simulink model "AUV_Model"  (R2023a)
settings: Solver=VariableStepAuto  StartTime=0.0  StopTime=300  FixedStep=0.5  RelTol=1e-3
InitFcn:
  | mdlWks = get_param(gcs,'ModelWorkspace');
  | a = getVariable(mdlWks,'a');
  | b = getVariable(mdlWks,'b');
  | c = getVariable(mdlWks,'c');
StopFcn:
  | figure(2)
  | plot3(Position_Data(1,1),Position_Data(1,2),Position_Data(1,3),'r*')
  | hold on
  | plot3(Position_Data(:,1),Position_Data(:,2),Position_Data(:,3));
  | plot3(Position_Data(end,1),Position_Data(end,2),Position_Data(end,3),'g*');
  | grid on
  | legend('Start Point','Trajectory','End Point')
model workspace (MAT data in the model file):
  a = 0
  b = 1
  c = 1
undefined symbols (not defined in the file or in its folder): sigbuilder_block
libraries: sharedtransform x6, vrlib x6, dspfdesign x6, sim3dlib x3, slpidlib x3, simulink x2, shared6dof x1, aerolibasang x1, aerolibnav x1, sim3dphyssensorlib x1
(part 1 of 2)
settings Model: Creator=yveerall  LastModifiedBy=kellthom
settings SolverCC: AlgebraicLoopSolver=TrustRegion
settings DataIOCC: ReturnWorkspaceOutputs=off
settings DebuggingCC: UnconnectedInputMsg=warning  UnconnectedOutputMsg=warning  UnconnectedLineMsg=warning  ArithmeticOperatorsInVariantConditions=warning
settings ModelReferenceCC: EnableRefExpFcnMdlSchedulingChecks=on
settings SFSimCC: CustomCodeUndefinedFunction=UseInterfaceOnly
settings RTWCC: DLArmComputeVersion=19.05

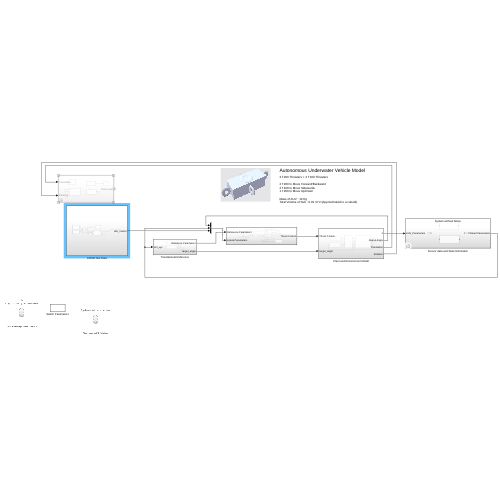
[thumbnail: Simulink's stored preview of the top-level diagram]
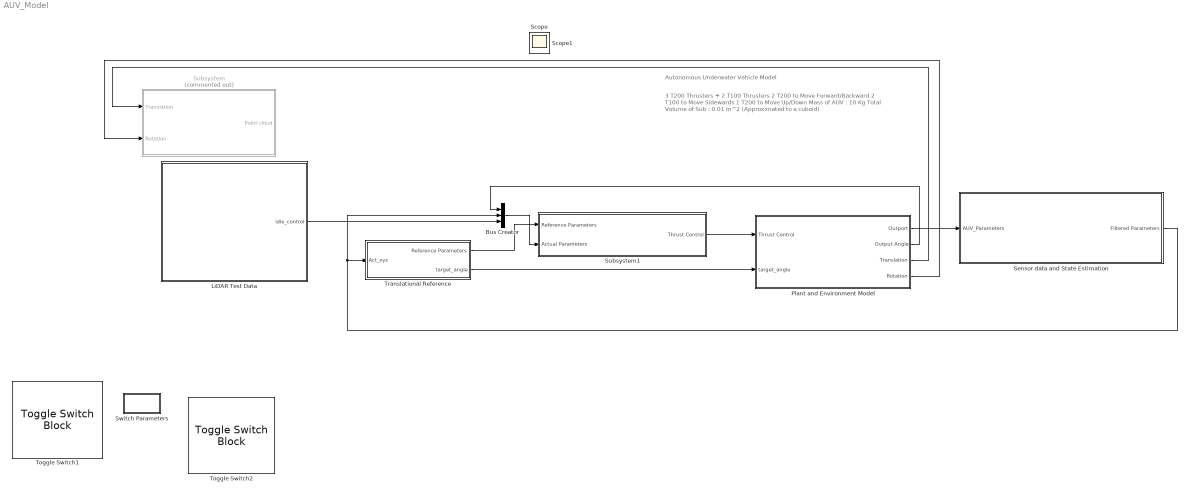
== system AUV_Model ==
  note: Autonomous Underwater Vehicle Model
  note: 3 T200 Thrusters + 2 T100 Thrusters
      |
      | 2 T200 to Move Forward/Backward
      | 2 T100 to Move Sidewards
      | 1 T200 to Move Up/Down
      |
      | Mass of AUV : 10 Kg
      | Total Volume of Sub : 0.01 m^2 (Approximated to a cuboid)
  Bus Creator : BusCreator  Inputs=3
  LiDAR Test Data : Subsystem
  Plant and Environment Model : Subsystem
  Sensor data and State Estimation : Subsystem  Variant=on
  Subsystem : Subsystem  Commented=on
  Subsystem1 : Subsystem
  Switch Parameters : Subsystem
      mask Display: text(0.5, 0.5, 'Switch Parameters', 'horizontalAlignment', 'center')
  Toggle Switch1 : ToggleSwitchBlock
      settings: Values={{'Low Fidelity Simulation', 'High Fidelity Simulation'}, [0 1]}
  Toggle Switch2 : ToggleSwitchBlock
      settings: Values={{'System with Noise', 'System without Noise'}, [0 1]}
  Translational Reference : Subsystem
  Scope : Scope
  Scope1 : Scope
  wires:
  Plant and Environment Model/1(Outport) -> Sensor data and State Estimation/1(AUV_Parameters)
  Sensor data and State Estimation/1(Filtered Parameters) -> Bus Creator/2, Translational Reference/1(Act_xyz)
  Translational Reference/2(target_angle) -> Plant and Environment Model/2(target_angle)
  Plant and Environment Model/4(Rotation) -> Subsystem/2(Rotation)
  Plant and Environment Model/3(Translation) -> Subsystem/1(Translation)
  Plant and Environment Model/2(Output Angle) -> Bus Creator/1
  Subsystem1/1(Thrust Control) -> Plant and Environment Model/1(Thrust Control)
  Translational Reference/1(Reference Parameters) -> Subsystem1/1(Reference Parameters)
  Bus Creator/1 -> Subsystem1/2(Actual Parameters)
  LiDAR Test Data/1(idle_control) -> Bus Creator/3

== system AUV_Model/LiDAR Test Data ==
  Clock : Clock
  Lidar control : MATLAB Function  TreatAsAtomicUnit=on
  MATLAB Function : MATLAB Function  TreatAsAtomicUnit=on
  MATLAB Function1 : MATLAB Function  TreatAsAtomicUnit=on
  Point Cloud Viewer : PointCloudViewer  FigPos=[161 681 522 480]
  Rate Transition : RateTransition  OutPortSampleTime=1
  Scope2 : Scope  NumInputPorts=2
  Switch : Switch  Criteria=u2 > Threshold  Threshold=9  SaturateOnIntegerOverflow=off  InputSameDT=off
  idle_control : Outport
  wires:
  Clock/1 -> Rate Transition/1
  Rate Transition/1 -> Switch/2, Lidar control/2(clock)
  Lidar control/2(state_o) -> Scope2/1
  MATLAB Function1/1(pcloud) -> Switch/3
  Switch/1 -> Point Cloud Viewer/1, Lidar control/1(point_cloud)
  Lidar control/1(idle_control) -> idle_control/1
  MATLAB Function/1(pcloud) -> Switch/1

== system AUV_Model/Plant and Environment Model ==
  Thrust Control : Inport
  target_angle : Inport  Port=2
  Combine Forces and Moments : Subsystem
  Dynamics solver : Subsystem
  Environmental Forces & Moments : Subsystem
  Propulsion Forces & Moments : Subsystem
  Outport : Outport  VectorParamsAs1DForOutWhenUnconnected=off
  Output Angle : Outport  Port=2
  Translation : Outport  Port=3  VectorParamsAs1DForOutWhenUnconnected=off
  Rotation : Outport  Port=4  VectorParamsAs1DForOutWhenUnconnected=off
  wires:
  Thrust Control/1 -> Propulsion Forces & Moments/1(Thrust Control In)
  Propulsion Forces & Moments/1(Propulsion Parameters) -> Combine Forces and Moments/1(Propulsion Parameters)
  Environmental Forces & Moments/1(Environment Parameters) -> Combine Forces and Moments/2(Hydrodynamic Force)
  Combine Forces and Moments/1(Total Force) -> Dynamics solver/1(Total Force)
  Combine Forces and Moments/2(Total Moment) -> Dynamics solver/2(Total Moment)
  Dynamics solver/1(AUV Data) -> Outport/1
  Dynamics solver/2(Internal Parameters) -> Environmental Forces & Moments/1(AOA_SideSlip)
  Dynamics solver/3(Output Angle) -> Output Angle/1
  target_angle/1 -> Dynamics solver/3(target angle)
  Dynamics solver/5(Rotation) -> Rotation/1
  Dynamics solver/4(Translation) -> Translation/1

== system AUV_Model/Sensor data and State Estimation ==
  AUV_Parameters : Inport
  System With Noise : Subsystem  VariantControl=b==0
  System without Noise : Subsystem  VariantControl=b==1
  Filtered Parameters : Outport  VectorParamsAs1DForOutWhenUnconnected=off

== system AUV_Model/Subsystem ==
  Translation : Inport
  Rotation : Inport  Port=2
  Constant : Constant  Value=[1 1 1]
  Simulation 3D Actor Transform Set : sim3dlib/Simulation 3D Actor Transform Set  Priority=-1  ActorTag=SimulinkActor1  NumberOfParts=1  CustNumOfParts=3  Translation=[0 0 0]  Rotation=[0 0 0]  Scale=[1 1 1]  Ts=-1  aMode=2
      settings: LibrarySourceBlock=vdynlib/Vehicle Scenarios/Sim3D/Sim3D Core/Simulation 3D Actor Transform Set
  Simulation 3D Camera Get : sim3dlib/Simulation 3D Camera Get  Priority=1  sensorTag=Sim3dSensor2  sensorId=2  sensorName=Sim3dSensor2  vehTagList={'Scene Origin'}  vehTag=Scene Origin  mountLoc=Origin  offsetFlag=off  tmountOffset=[0, 0, 0]  rmountOffset=[0, 0, 0]  HorizontalResolution=1280  VerticalResolution=720  HorizontalFOV=60  SampleTime=-1  mountPoint=[0 0 0]  mountOrientation=[0 0 0]  aMode=2  ID=2
      settings: LibrarySourceBlock=vdynlib/Vehicle Scenarios/Sim3D/Sim3D Core/Simulation 3D Camera Get
  Simulation 3D Lidar : sim3dphyssensorlib/Simulation 3D Lidar  Priority=1  sensorTag=Sim3dSensor1  sensorId=1  sensorName=Sim3dSensor1  vehTagList={'Scene Origin'}  vehTag=Scene Origin  mountLoc=Origin  offsetFlag=off  tmountOffset=[0, 0, 0]  rmountOffset=[0, 0, 0]  DetectionRange=120  RangeResolution=0.002  VerticalFOV=40  VerticalResolution=1.25  HorizontalFOV=360  HorizontalResolution=0.16  DistanceOutportEnabled=off  ReflectivityOutportEnabled=off  SemanticOutportEnabled=off  TransformOutportEnabled=off  SampleTime=-1  mountPoint=[0 0 0]  mountOrientation=[0 0 0]  aMode=3  ID=1
      settings: LibrarySourceBlock=drivingsim3d/Simulation 3D Lidar
  Simulation 3D Scene Configuration : sim3dlib/Simulation 3D Scene Configuration  Priority=0  ProjectFormat=Default Scenes  SceneDesc=Straight road  ProjectName=/share/pkg.7/matlab/2023a/install/toolbox/shared/sim3d_projects/automotive_project/UE4/LinuxNoEditor/AutoVrtlEnv.sh  ScenePath=/Game/Maps/HwStrght  EnableOpenDRIVE=off  vehTagList={'Scene Origin'}  vehTag=Scene Origin  OpVisEn=off  Ts=.02  EnableWindow=on  EnableRemoteAccess=off  EnableWeather=off  SunAltitude=40.0  SunAzimuth=90  clouds=10  wind=1  fog=0  rain=0  EnableGeospatial=off  OriginHeight=200  OriginLatitude=40.744652  OriginLongitude=-73.988864  MapStyle=Aerial  AdditionalAssetIDs=[]  UseAdvancedSunSky=off  SolarTime=11  TimeZone=-5  Day=21  Month=9  Year=2022  UseDaylightSavingTime=on  DSTStartDay=10  DSTStartMonth=3  DSTEndDay=3  DSTEndMonth=11  DSTSwitchHour=2  sensorTag=MainCamera1  sensorId=1  sensorName=MainCamera1  mountLoc=Origin  offsetFlag=off  tmountOffset=[0, 0, 0]  rmountOffset=[0, 0, 0]  HorizontalResolution=1280  VerticalResolution=720  HorizontalFOV=60  mountPoint=[0 0 0]  mountOrientation=[0 0 0]  aMode=2  ID=1  GeoTrigger=Inactive
      settings: LibrarySourceBlock=vdynlib/Vehicle Scenarios/Sim3D/Sim3D Core/Simulation 3D Scene Configuration
  Video Viewer : VideoViewer  FigPos=[622 528 418 304]
  Point cloud : Outport
  wires:
  Simulation 3D Lidar/1 -> Point cloud/1
  Simulation 3D Camera Get/1 -> Video Viewer/1
  Constant/1 -> Simulation 3D Actor Transform Set/3
  Translation/1 -> Simulation 3D Actor Transform Set/1
  Rotation/1 -> Simulation 3D Actor Transform Set/2

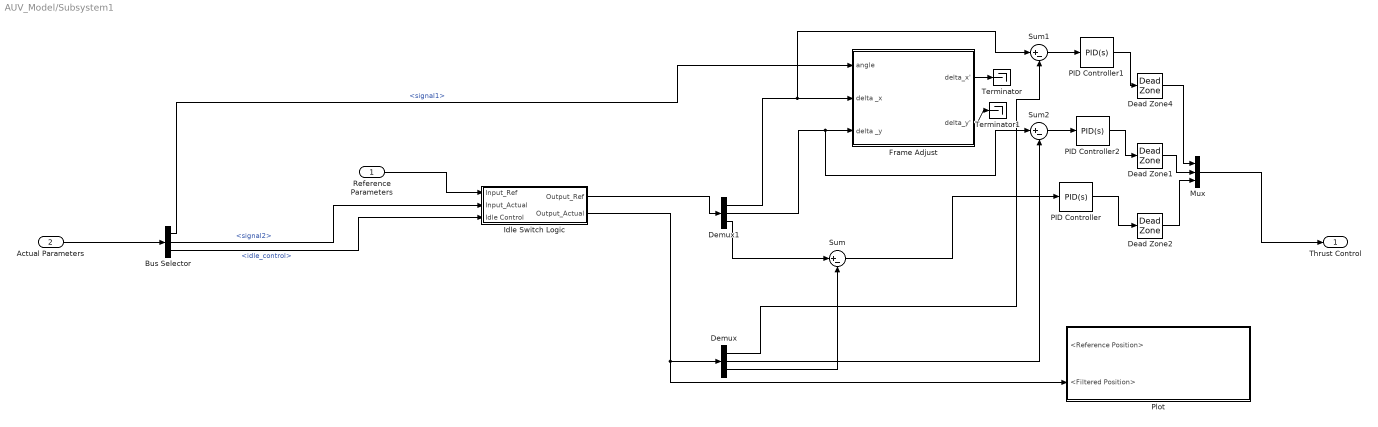
== system AUV_Model/Subsystem1 ==
  Reference Parameters : Inport
  Actual Parameters : Inport  Port=2
  Bus Selector : BusSelector  OutputSignals=signal1,signal2,idle_control
  Dead Zone1 : DeadZone  LowerValue=-0.05  UpperValue=+0.05
  Dead Zone2 : DeadZone  LowerValue=-0.05  UpperValue=+0.05
  Dead Zone4 : DeadZone  LowerValue=-0.05  UpperValue=+0.05
  Demux : Demux  Outputs=3
  Demux1 : Demux  Outputs=3
  Frame Adjust : Subsystem
  Idle Switch Logic : Subsystem
  Mux : Mux  Inputs=3
  PID Controller : slpidlib/PID Controller  Controller=PID  Form=Parallel  TimeDomain=Continuous-time  UseExternalTs=off  SampleTime=-1  IntegratorMethod=Forward Euler  FilterMethod=Forward Euler  ControllerParametersSource=internal  P=-0.0440831016133051  I=-0.00046335965727533  UseKiTs=off  D=-0.931852208113014  N=205.904485551143  UseFilter=on  TunerSelectOption=Transfer Function Based (PID Tuner App)  InitialConditionSource=internal  InitialConditionForIntegrator=0  InitialConditionForFilter=0  DifferentiatorICPrevScaledInput=0  ExternalReset=none  TrackingMode=off  Kt=1  LimitOutput=off  SatLimitsSource=internal  UpperSaturationLimit=inf  LowerSaturationLimit=-inf  LinearizeAsGain=on  AntiWindupMode=none  Kb=1  LimitIntegrator=off  UpperIntegratorSaturationLimit=inf  LowerIntegratorSaturationLimit=-inf  POutMin=[]  POutMax=[]  IOutMin=[]  IOutMax=[]  DOutMin=[]  DOutMax=[]  NOutMin=[]  NOutMax=[]  SumOutMin=[]  SumOutMax=[]  SaturationOutMin=[]  SaturationOutMax=[]  PParamMin=[]  PParamMax=[]  IParamMin=[]  IParamMax=[]  DParamMin=[]  DParamMax=[]  NParamMin=[]  NParamMax=[]  KbParamMin=[]  KbParamMax=[]  KtParamMin=[]  KtParamMax=[]  KbOutMin=[]  KbOutMax=[]  KtOutMin=[]  KtOutMax=[]  IntegratorOutMin=[]  IntegratorOutMax=[]  FilterOutMin=[]  FilterOutMax=[]  SumI1OutMin=[]  SumI1OutMax=[]  SumI2OutMin=[]  SumI2OutMax=[]  SumI3OutMin=[]  SumI3OutMax=[]  SumI4OutMin=[]  SumI4OutMax=[]  SumDOutMin=[]  SumDOutMax=[]  DifferentiatorOutMin=[]  DifferentiatorOutMax=[]  FilterDiffOutCoefMin=[]  FilterDiffOutCoefMax=[]  ReciprocalOutMin=[]  ReciprocalOutMax=[]  SumDenOutMin=[]  SumDenOutMax=[]  SumNumOutMin=[]  SumNumOutMax=[]  DivideOutMin=[]  DivideOutMax=[]  UdiffTsProdOutMin=[]  UdiffTsProdOutMax=[]  NTsProdOutMin=[]  NTsProdOutMax=[]  UintegralTsProdOutMin=[]  UintegralTsProdOutMax=[]  UngainTsProdOutMin=[]  UngainTsProdOutMax=[]  ClampingZeroOutDataTypeStr=Inherit: Inherit via back propagation  ClampingZeroOutMin=[]  ClampingZeroOutMax=[]  FilterDenConstantOutDataTypeStr=Inherit: Inherit via back propagation  FilterDenConstantOutMin=[]  FilterDenConstantOutMax=[]  PCopyOutDataTypeStr=Inherit: Inherit via back propagation  PCopyOutMin=[]  PCopyOutMax=[]  NCopyOutDataTypeStr=Inherit: Inherit via back propagation  NCopyOutMin=[]  NCopyOutMax=[]  IntegratorContinuousStateAttributes=''  IntegratorStateMustResolveToSignalObject=off  IntegratorRTWStateStorageClass=Auto  FilterContinuousStateAttributes=''  FilterStateMustResolveToSignalObject=off  FilterRTWStateStorageClass=Auto  ParallelPVariant=InternalParameters  IdealPVariant=Disabled  IVariant=InternalParameters  DVariant=InternalParameters  IntegratorVariant=Continuous  SatVariant=Disabled  AWVariant=Passthrough  PCopyVariant=Disabled  TRVariant=Disabled  FdbkBlocksVariant=Forward  IdealPFdbkVariant=Disabled  SatFdbkVariant=Disabled  DerivativeFilterVariant=ContFilter  NVariant=InternalParameters  NCopyVariant=Disabled  FilterICVariant=InternalICsFilter  IntegratorICVariant=InternalICs  ExternalResetVariant=Disabled  TRSumVariant=Passthrough  SumFdbkVariant=Disabled  SumVariant=Sum_PID  TsampFilterVariant=InternalTs  TsampNgainVariant=Passthrough  TsampIntegralVariant=Disabled_SignalSpec  ExternalSaturationOutDataTypeStr=Inherit: Same as second input
  PID Controller1 : slpidlib/PID Controller  Controller=PID  Form=Parallel  TimeDomain=Continuous-time  UseExternalTs=off  SampleTime=-1  IntegratorMethod=Forward Euler  FilterMethod=Forward Euler  ControllerParametersSource=internal  P=0.0352909553215239  I=0.000468513300704798  UseKiTs=off  D=0.59064410837381  N=260.062804539004  UseFilter=on  TunerSelectOption=Transfer Function Based (PID Tuner App)  InitialConditionSource=internal  InitialConditionForIntegrator=0  InitialConditionForFilter=0  DifferentiatorICPrevScaledInput=0  ExternalReset=none  TrackingMode=off  Kt=1  LimitOutput=off  SatLimitsSource=internal  UpperSaturationLimit=inf  LowerSaturationLimit=-inf  LinearizeAsGain=on  AntiWindupMode=none  Kb=1  LimitIntegrator=off  UpperIntegratorSaturationLimit=inf  LowerIntegratorSaturationLimit=-inf  POutMin=[]  POutMax=[]  IOutMin=[]  IOutMax=[]  DOutMin=[]  DOutMax=[]  NOutMin=[]  NOutMax=[]  SumOutMin=[]  SumOutMax=[]  SaturationOutMin=[]  SaturationOutMax=[]  PParamMin=[]  PParamMax=[]  IParamMin=[]  IParamMax=[]  DParamMin=[]  DParamMax=[]  NParamMin=[]  NParamMax=[]  KbParamMin=[]  KbParamMax=[]  KtParamMin=[]  KtParamMax=[]  KbOutMin=[]  KbOutMax=[]  KtOutMin=[]  KtOutMax=[]  IntegratorOutMin=[]  IntegratorOutMax=[]  FilterOutMin=[]  FilterOutMax=[]  SumI1OutMin=[]  SumI1OutMax=[]  SumI2OutMin=[]  SumI2OutMax=[]  SumI3OutMin=[]  SumI3OutMax=[]  SumI4OutMin=[]  SumI4OutMax=[]  SumDOutMin=[]  SumDOutMax=[]  DifferentiatorOutMin=[]  DifferentiatorOutMax=[]  FilterDiffOutCoefMin=[]  FilterDiffOutCoefMax=[]  ReciprocalOutMin=[]  ReciprocalOutMax=[]  SumDenOutMin=[]  SumDenOutMax=[]  SumNumOutMin=[]  SumNumOutMax=[]  DivideOutMin=[]  DivideOutMax=[]  UdiffTsProdOutMin=[]  UdiffTsProdOutMax=[]  NTsProdOutMin=[]  NTsProdOutMax=[]  UintegralTsProdOutMin=[]  UintegralTsProdOutMax=[]  UngainTsProdOutMin=[]  UngainTsProdOutMax=[]  ClampingZeroOutDataTypeStr=Inherit: Inherit via back propagation  ClampingZeroOutMin=[]  ClampingZeroOutMax=[]  FilterDenConstantOutDataTypeStr=Inherit: Inherit via back propagation  FilterDenConstantOutMin=[]  FilterDenConstantOutMax=[]  PCopyOutDataTypeStr=Inherit: Inherit via back propagation  PCopyOutMin=[]  PCopyOutMax=[]  NCopyOutDataTypeStr=Inherit: Inherit via back propagation  NCopyOutMin=[]  NCopyOutMax=[]  IntegratorContinuousStateAttributes=''  IntegratorStateMustResolveToSignalObject=off  IntegratorRTWStateStorageClass=Auto  FilterContinuousStateAttributes=''  FilterStateMustResolveToSignalObject=off  FilterRTWStateStorageClass=Auto  ParallelPVariant=InternalParameters  IdealPVariant=Disabled  IVariant=InternalParameters  DVariant=InternalParameters  IntegratorVariant=Continuous  SatVariant=Disabled  AWVariant=Passthrough  PCopyVariant=Disabled  TRVariant=Disabled  FdbkBlocksVariant=Forward  IdealPFdbkVariant=Disabled  SatFdbkVariant=Disabled  DerivativeFilterVariant=ContFilter  NVariant=InternalParameters  NCopyVariant=Disabled  FilterICVariant=InternalICsFilter  IntegratorICVariant=InternalICs  ExternalResetVariant=Disabled  TRSumVariant=Passthrough  SumFdbkVariant=Disabled  SumVariant=Sum_PID  TsampFilterVariant=InternalTs  TsampNgainVariant=Passthrough  TsampIntegralVariant=Disabled_SignalSpec  ExternalSaturationOutDataTypeStr=Inherit: Same as second input
  PID Controller2 : slpidlib/PID Controller  Controller=PID  Form=Parallel  TimeDomain=Continuous-time  UseExternalTs=off  SampleTime=-1  IntegratorMethod=Forward Euler  FilterMethod=Forward Euler  ControllerParametersSource=internal  P=0.172975950646219  I=0.00387308418128247  UseKiTs=off  D=1.71646711354372  N=438.622536688858  UseFilter=on  TunerSelectOption=Transfer Function Based (PID Tuner App)  InitialConditionSource=internal  InitialConditionForIntegrator=0  InitialConditionForFilter=0  DifferentiatorICPrevScaledInput=0  ExternalReset=none  TrackingMode=off  Kt=1  LimitOutput=off  SatLimitsSource=internal  UpperSaturationLimit=inf  LowerSaturationLimit=-inf  LinearizeAsGain=on  AntiWindupMode=none  Kb=1  LimitIntegrator=off  UpperIntegratorSaturationLimit=inf  LowerIntegratorSaturationLimit=-inf  POutMin=[]  POutMax=[]  IOutMin=[]  IOutMax=[]  DOutMin=[]  DOutMax=[]  NOutMin=[]  NOutMax=[]  SumOutMin=[]  SumOutMax=[]  SaturationOutMin=[]  SaturationOutMax=[]  PParamMin=[]  PParamMax=[]  IParamMin=[]  IParamMax=[]  DParamMin=[]  DParamMax=[]  NParamMin=[]  NParamMax=[]  KbParamMin=[]  KbParamMax=[]  KtParamMin=[]  KtParamMax=[]  KbOutMin=[]  KbOutMax=[]  KtOutMin=[]  KtOutMax=[]  IntegratorOutMin=[]  IntegratorOutMax=[]  FilterOutMin=[]  FilterOutMax=[]  SumI1OutMin=[]  SumI1OutMax=[]  SumI2OutMin=[]  SumI2OutMax=[]  SumI3OutMin=[]  SumI3OutMax=[]  SumI4OutMin=[]  SumI4OutMax=[]  SumDOutMin=[]  SumDOutMax=[]  DifferentiatorOutMin=[]  DifferentiatorOutMax=[]  FilterDiffOutCoefMin=[]  FilterDiffOutCoefMax=[]  ReciprocalOutMin=[]  ReciprocalOutMax=[]  SumDenOutMin=[]  SumDenOutMax=[]  SumNumOutMin=[]  SumNumOutMax=[]  DivideOutMin=[]  DivideOutMax=[]  UdiffTsProdOutMin=[]  UdiffTsProdOutMax=[]  NTsProdOutMin=[]  NTsProdOutMax=[]  UintegralTsProdOutMin=[]  UintegralTsProdOutMax=[]  UngainTsProdOutMin=[]  UngainTsProdOutMax=[]  ClampingZeroOutDataTypeStr=Inherit: Inherit via back propagation  ClampingZeroOutMin=[]  ClampingZeroOutMax=[]  FilterDenConstantOutDataTypeStr=Inherit: Inherit via back propagation  FilterDenConstantOutMin=[]  FilterDenConstantOutMax=[]  PCopyOutDataTypeStr=Inherit: Inherit via back propagation  PCopyOutMin=[]  PCopyOutMax=[]  NCopyOutDataTypeStr=Inherit: Inherit via back propagation  NCopyOutMin=[]  NCopyOutMax=[]  IntegratorContinuousStateAttributes=''  IntegratorStateMustResolveToSignalObject=off  IntegratorRTWStateStorageClass=Auto  FilterContinuousStateAttributes=''  FilterStateMustResolveToSignalObject=off  FilterRTWStateStorageClass=Auto  ParallelPVariant=InternalParameters  IdealPVariant=Disabled  IVariant=InternalParameters  DVariant=InternalParameters  IntegratorVariant=Continuous  SatVariant=Disabled  AWVariant=Passthrough  PCopyVariant=Disabled  TRVariant=Disabled  FdbkBlocksVariant=Forward  IdealPFdbkVariant=Disabled  SatFdbkVariant=Disabled  DerivativeFilterVariant=ContFilter  NVariant=InternalParameters  NCopyVariant=Disabled  FilterICVariant=InternalICsFilter  IntegratorICVariant=InternalICs  ExternalResetVariant=Disabled  TRSumVariant=Passthrough  SumFdbkVariant=Disabled  SumVariant=Sum_PID  TsampFilterVariant=InternalTs  TsampNgainVariant=Passthrough  TsampIntegralVariant=Disabled_SignalSpec  ExternalSaturationOutDataTypeStr=Inherit: Same as second input
  Plot : Subsystem
  Sum : Sum  Inputs=|+-
  Sum1 : Sum  Inputs=|+-
  Sum2 : Sum  Inputs=|+-
  Terminator : Terminator
  Terminator1 : Terminator
  Thrust Control : Outport  VectorParamsAs1DForOutWhenUnconnected=off
  wires:
  Dead Zone1/1 -> Mux/2
  PID Controller/1 -> Dead Zone2/1
  Idle Switch Logic/1(Output_Ref) -> Demux1/1
  Demux/1 -> Sum1/2
  Reference Parameters/1 -> Idle Switch Logic/1(Input_Ref)
  Demux1/3 -> Sum/1
  Demux1/1 -> Sum1/1, Frame Adjust/2(delta _x)
  Frame Adjust/1(delta_x') -> Terminator/1
  Mux/1 -> Thrust Control/1
  Actual Parameters/1 -> Bus Selector/1
  Sum1/1 -> PID Controller1/1
  Dead Zone4/1 -> Mux/1
  Sum/1 -> PID Controller/1
  Bus Selector/1 -> Frame Adjust/1(angle)  "<signal1>"
  Demux/2 -> Sum2/2
  Frame Adjust/2(delta_y') -> Terminator1/1
  Bus Selector/2 -> Idle Switch Logic/2(Input_Actual)  "<signal2>"
  Idle Switch Logic/2(Output_Actual) -> Plot/2(<Filtered Position>), Demux/1
  PID Controller2/1 -> Dead Zone1/1
  Demux1/2 -> Sum2/1, Frame Adjust/3(delta _y)
  Demux/3 -> Sum/2
  Dead Zone2/1 -> Mux/3
  PID Controller1/1 -> Dead Zone4/1
  Sum2/1 -> PID Controller2/1
  Bus Selector/3 -> Idle Switch Logic/3(Idle Control)  "<idle_control>"

== system AUV_Model/Switch Parameters ==
  Constant : Constant  Value=a
  Constant1 : Constant  Value=b
  Constant2 : Constant  Value=c
  Terminator1 : Terminator
  Terminator2 : Terminator
  Terminator3 : Terminator
  wires:
  Constant/1 -> Terminator1/1
  Constant1/1 -> Terminator2/1
  Constant2/1 -> Terminator3/1

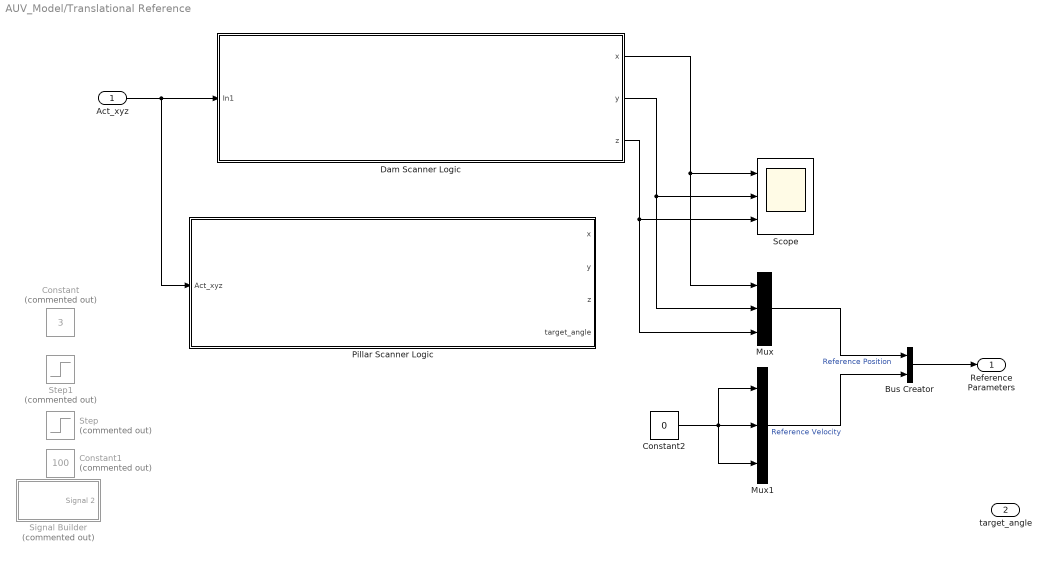
== system AUV_Model/Translational Reference ==
  Act_xyz : Inport
  Bus Creator : BusCreator  Inputs=2
  Constant : Constant  Commented=on  Value=3
  Constant1 : Constant  Commented=on  Value=100
  Constant2 : Constant  Value=0
  Dam Scanner Logic : Subsystem
  Mux : Mux  Inputs=3
  Mux1 : Mux  Inputs=3
  Pillar Scanner Logic : Subsystem
  Scope : Scope  NumInputPorts=3
  Signal Builder : Subsystem  Tag=STV Subsys  Commented=on  LoadFcn=sigbuilder_block('load');  StartFcn=sigbuilder_block('start');  StopFcn=sigbuilder_block('stop');  ClipboardFcn=sigbuilder_block('clipboard');  mask(Sigbuilder block){tuvar=[0:10]}
      mask help: Simulink:masks:SigbuilderBlock_MD
      mask init:
      | if ~strcmp(get_param(bdroot(gcbh),'SimulationStatus'),'stopped') tuvar = sigbuilder_block('maskInit'); end
      settings: CopyFcn=sigbuilder_block('copy');  DeleteFcn=sigbuilder_block('delete');  ModelCloseFcn=sigbuilder_block('modelClose');  PreSaveFcn=sigbuilder_block('preSave');  PauseFcn=sigbuilder_block('pause');  ContinueFcn=sigbuilder_block('continue');  NameChangeFcn=sigbuilder_block('namechange');  OpenFcn=sigbuilder_block('open',[-82.6105 -97.7684 948.884 357.726 ]);  CloseFcn=sigbuilder_block('close');
      mask Display: plot(0, 0, 100, 100,[2, 2, 32, 32, 2], [68, 8, 8, 68, 68],[32, 2], [38, 38], [32, 19, 2],[53, 60, 44], [32, 17, 17, 2],[16, 16, 31, 31]);txt = getActiveGroup(gcbh);text(2, 100, txt,'verticalAlignment', 'top');
  Step : Step  Commented=on  Time=30  Before=0.2  After=0  SampleTime=0
  Step1 : Step  Commented=on  Time=150  Before=10  After=5  SampleTime=0
  Reference Parameters : Outport  VectorParamsAs1DForOutWhenUnconnected=off
  target_angle : Outport  Port=2  VectorParamsAs1DForOutWhenUnconnected=off
  wires:
  Mux/1 -> Bus Creator/1  "Reference Position"
  Mux1/1 -> Bus Creator/2  "Reference Velocity"
  Bus Creator/1 -> Reference Parameters/1
  Constant2/1 -> Mux1/1, Mux1/3, Mux1/2
  Act_xyz/1 -> Pillar Scanner Logic/1(Act_xyz), Dam Scanner Logic/1(In1)
  Dam Scanner Logic/1(x) -> Mux/1, Scope/1
  Dam Scanner Logic/2(y) -> Mux/2, Scope/2
  Dam Scanner Logic/3(z) -> Scope/3, Mux/3

== system AUV_Model/Plant and Environment Model/Combine Forces and Moments ==
  Propulsion Parameters : Inport
  Hydrodynamic Force : Inport  Port=2
  Bus Selector : BusSelector  OutputSignals=PropForce,PropMoment
  Bus Selector1 : BusSelector  OutputSignals=LDForce,HSForce,HS Moment
  Saturation : Saturate  UpperLimit=600  LowerLimit=-600
  Saturation1 : Saturate  UpperLimit=600  LowerLimit=-600
  Sum : Sum  Inputs=+++
  Sum1 : Sum  Inputs=|++
  Total Force : Outport  VectorParamsAs1DForOutWhenUnconnected=off
  Total Moment : Outport  Port=2  VectorParamsAs1DForOutWhenUnconnected=off
  wires:
  Bus Selector1/3 -> Sum1/2  "<HS Moment>"
  Bus Selector/2 -> Sum1/1  "<PropMoment>"
  Sum/1 -> Saturation/1
  Sum1/1 -> Total Moment/1
  Saturation1/1 -> Sum/2
  Saturation/1 -> Total Force/1
  Propulsion Parameters/1 -> Bus Selector/1
  Hydrodynamic Force/1 -> Bus Selector1/1
  Bus Selector/1 -> Sum/1  "<PropForce>"
  Bus Selector1/1 -> Saturation1/1  "<LDForce>"
  Bus Selector1/2 -> Sum/3  "<HSForce>"

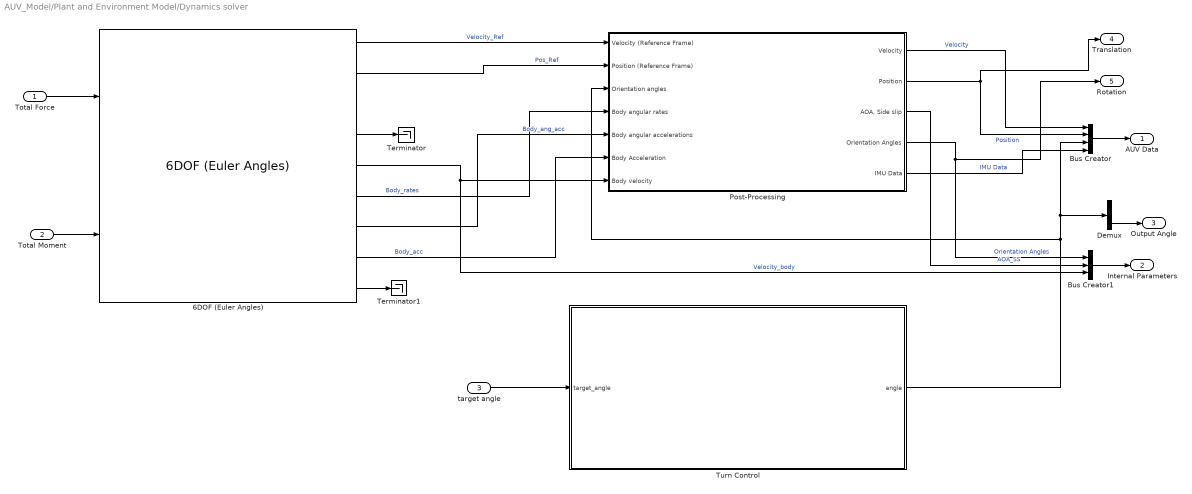
== system AUV_Model/Plant and Environment Model/Dynamics solver ==
  Total Force : Inport
  Total Moment : Inport  Port=2
  target angle : Inport  Port=3
  6DOF (Euler Angles) : shared6dof/6DOF (Euler Angles)  units=Metric (MKS)  mtype=Fixed  rep=Euler Angles  xme_0=[0.01 .01 .01]  Vm_0=[0.01 0.01 0.001]  eul_0=[0.001 0.001 0.001]  pm_0=[0.001 0.001 0.001]  mass_0=10  mass_e=0.5  mass_f=2.0  inertia=10*eye(3)  inertia_e=eye(3)  inertia_f=2*eye(3)  k_quat=1.0  vre_flag=on  abi_flag=on  aMode=0  xme_statename=''  Vm_statename=''  eul_statename=''  quat_statename=''  pm_statename=''  mass_statename=''
  Bus Creator : BusCreator  Inputs=4
  Bus Creator1 : BusCreator  Inputs=3
  Demux : Demux  Outputs=3
  Post-Processing : Subsystem
  Terminator : Terminator
  Terminator1 : Terminator
  Turn Control : Subsystem
  AUV Data : Outport  VectorParamsAs1DForOutWhenUnconnected=off
  Internal Parameters : Outport  Port=2  VectorParamsAs1DForOutWhenUnconnected=off
  Output Angle : Outport  Port=3
  Translation : Outport  Port=4  VectorParamsAs1DForOutWhenUnconnected=off
  Rotation : Outport  Port=5  VectorParamsAs1DForOutWhenUnconnected=off
  wires:
  6DOF (Euler Angles)/6 -> Post-Processing/4(Body angular rates)  "Body_rates"
  Post-Processing/3("AOA, Side slip") -> Bus Creator1/2  "AOA_SS"
  6DOF (Euler Angles)/8 -> Post-Processing/6(Body Acceleration)  "Body_acc"
  Post-Processing/2(" Position") -> Bus Creator/2, Translation/1  "Position"
  6DOF (Euler Angles)/7 -> Post-Processing/5(Body angular accelerations)  "Body_ang_acc"
  6DOF (Euler Angles)/2 -> Post-Processing/2(Position (Reference Frame))  "Pos_Ref"
  Post-Processing/1(Velocity) -> Bus Creator/1  "Velocity"
  6DOF (Euler Angles)/1 -> Post-Processing/1(Velocity (Reference Frame))  "Velocity_Ref"
  6DOF (Euler Angles)/5 -> Bus Creator1/3, Post-Processing/7(Body velocity)  "Velocity_body"
  Post-Processing/4(Orientation Angles) -> Rotation/1, Bus Creator1/1  "Orientation Angles"
  Post-Processing/5(IMU Data) -> Bus Creator/4  "IMU Data"
  Total Force/1 -> 6DOF (Euler Angles)/1
  Total Moment/1 -> 6DOF (Euler Angles)/2
  Bus Creator/1 -> AUV Data/1
  Bus Creator1/1 -> Internal Parameters/1
  6DOF (Euler Angles)/4 -> Terminator/1
  6DOF (Euler Angles)/9 -> Terminator1/1
  Turn Control/1(angle) -> Demux/1, Bus Creator/3, Post-Processing/3(Orientation angles)
  Demux/3 -> Output Angle/1
  target angle/1 -> Turn Control/1(target_angle)

== system AUV_Model/Plant and Environment Model/Environmental Forces & Moments ==
  AOA_SideSlip : Inport
  Bus Creator : BusCreator  Inputs=3
  Bus Selector : BusSelector  OutputSignals=Velocity_body,AOA_SS,Orientation Angles
  Hydrodynamic Forces : Subsystem  Variant=on
  Hydrostatic Forces : Subsystem
  Environment Parameters : Outport  VectorParamsAs1DForOutWhenUnconnected=off
  wires:
  Hydrodynamic Forces/1("Force due to Lift, Drag") -> Bus Creator/1  "LDForce"
  Hydrostatic Forces/1(Hydrostatic Force) -> Bus Creator/2  "HSForce"
  Hydrostatic Forces/2(Hydrostatic Moment) -> Bus Creator/3  "HS Moment"
  Bus Creator/1 -> Environment Parameters/1
  AOA_SideSlip/1 -> Bus Selector/1
  Bus Selector/1 -> Hydrodynamic Forces/1("Submarine Velocity (Body Axis) ")  "<Velocity_body>"
  Bus Selector/2 -> Hydrodynamic Forces/2("AOA, Side Slip")  "<AOA_SS>"
  Bus Selector/3 -> Hydrostatic Forces/1(In1)  "<Orientation Angles>"

== system AUV_Model/Plant and Environment Model/Propulsion Forces & Moments ==
  Thrust Control In : Inport
  Bus Creator : BusCreator  Inputs=2
  Force and moments due to Thrust : Subsystem
  Input commands to Thrust : Subsystem
  Propulsion Parameters : Outport  VectorParamsAs1DForOutWhenUnconnected=off
  wires:
  Input commands to Thrust/1(Thrust values) -> Force and moments due to Thrust/1(Thrust Inputs)
  Thrust Control In/1 -> Input commands to Thrust/1(Thrust Control Inputs)
  Force and moments due to Thrust/1(Propulsion Force) -> Bus Creator/1  "PropForce"
  Force and moments due to Thrust/2(Propulsion Moment) -> Bus Creator/2  "PropMoment"
  Bus Creator/1 -> Propulsion Parameters/1

== system AUV_Model/Sensor data and State Estimation/System With Noise ==
  AUV_Parameters : Inport
  " Sensor (IMU)" : Subsystem
  Internal filter : Subsystem
  Filtered Parameters : Outport  VectorParamsAs1DForOutWhenUnconnected=off
  wires:
  AUV_Parameters/1 -> " Sensor (IMU)"/1(IMU Inputs)
  Internal filter/1(Filtered Parameters) -> Filtered Parameters/1
  " Sensor (IMU)"/1(IMU Measurements) -> Internal filter/1(Accel)

== system AUV_Model/Sensor data and State Estimation/System without Noise ==
  AUV_Parameters : Inport
  Bus Creator : BusCreator  Inputs=2
  Bus Selector : BusSelector  OutputSignals=Position,Velocity
  Gain : Gain
  Gain1 : Gain
  Filtered Parameters : Outport  VectorParamsAs1DForOutWhenUnconnected=off
  wires:
  Bus Creator/1 -> Filtered Parameters/1
  Bus Selector/2 -> Gain1/1  "<Velocity>"
  Bus Selector/1 -> Gain/1  "<Position>"
  Gain1/1 -> Bus Creator/2  "Filtered Velocity"
  Gain/1 -> Bus Creator/1  "Filtered Position"
  AUV_Parameters/1 -> Bus Selector/1

== system AUV_Model/Subsystem1/Frame Adjust ==
  note: Our mode supports rotations in the xy plane, so it is necessary to have this logic to adjust the reference position with repect to the angle of the primed frame. This block is currently unused becuase turning will not be utilized in the dynamic solver.
  angle : Inport
  delta _x : Inport  Port=2
  delta _y : Inport  Port=3
  Constant1 : Constant  Value=2*pi  VectorParams1D=off
  Cosine : simulink/Lookup Tables/Cosine  Formula=cos(2*pi*u)  NumDataPoints=(2^5)+1  OutputWordLength=16  InternalRulePriority=Speed
  Divide : Product  Inputs=*/
  Product{,1..3} (4 alike) : Product
  Sine : simulink/Lookup Tables/Sine  Formula=sin(2*pi*u)  NumDataPoints=(2^5)+1  OutputWordLength=16  InternalRulePriority=Speed
  Sum3 : Sum  Inputs=|+-
  Sum4 : Sum  Inputs=|++
  delta_x' : Outport
  delta_y' : Outport  Port=2
  wires:
  Product3/1 -> Sum4/2
  delta _x/1 -> Product/2, Product2/1
  Product2/1 -> Sum4/1
  Product/1 -> Sum3/1
  Sine/1 -> Product2/2, Product1/2
  Product1/1 -> Sum3/2
  Sum3/1 -> delta_x'/1
  delta _y/1 -> Product1/1, Product3/1
  Cosine/1 -> Product/1, Product3/2
  Sum4/1 -> delta_y'/1
  Constant1/1 -> Divide/2
  angle/1 -> Divide/1
  Divide/1 -> Sine/1, Cosine/1

== system AUV_Model/Subsystem1/Idle Switch Logic ==
  note: When the switch is set to "proceed", the normal reference and actual position are passed.
      | When it is set to "idle", the reference is set to the postion when the switch was flipped.  This helps minimize the effect of noise and accumulation of drift.  11/2/24 Thomas
  Input_Ref : Inport
  Input_Actual : Inport  Port=2
  Idle Control : Inport  Port=3
  Bus Selector : BusSelector  OutputSignals=Filtered Position
  Bus Selector1 : BusSelector  OutputSignals=Reference Position
  Constant : Constant
  Switch : Switch  Criteria=u2 > Threshold  SaturateOnIntegerOverflow=off  InputSameDT=off
  Switch1 : Switch  Criteria=u2 > Threshold  SaturateOnIntegerOverflow=off  InputSameDT=off
  Output_Ref : Outport
  Output_Actual : Outport  Port=2
  wires:
  Bus Selector/1 -> Output_Actual/1, Switch1/1  "<Filtered Position>"
  Bus Selector1/1 -> Switch/1  "<Reference Position>"
  Input_Actual/1 -> Bus Selector/1
  Switch/1 -> Output_Ref/1
  Switch1/1 -> Switch1/3, Switch/3
  Input_Ref/1 -> Bus Selector1/1
  Constant/1 -> Switch1/2, Switch/2

== system AUV_Model/Subsystem1/Plot ==
  <Reference Position> : Inport
  <Filtered Position> : Inport  Port=2
  Demux2 : Demux  Outputs=3
  Demux3 : Demux  Outputs=3
  Mux1 : Mux  Inputs=2
  Mux2 : Mux  Inputs=2
  Mux3 : Mux  Inputs=2
  Scope : Scope  NumInputPorts=3
  wires:
  Mux3/1 -> Scope/3
  Demux3/1 -> Mux1/2
  Demux3/2 -> Mux2/2
  Demux2/3 -> Mux3/1
  Mux2/1 -> Scope/2
  Mux1/1 -> Scope/1
  Demux2/2 -> Mux2/1
  Demux2/1 -> Mux1/1
  Demux3/3 -> Mux3/2
  <Reference Position>/1 -> Demux2/1
  <Filtered Position>/1 -> Demux3/1

== system AUV_Model/Translational Reference/Dam Scanner Logic ==
  note: This logic takes in some dam parameters and the actual position of the robot (provided by the dynamic solver) and updates the reference position to make the robot move along the dam. 11/2/2024 Thomas
  In1 : Inport
  Bus Selector : BusSelector  OutputSignals=Filtered Position
  Constant4 : Constant  Value=100
  Constant5 : Constant  Value=10
  Constant6 : Constant  Value=5
  Delay : Delay  DelayLength=1  InitialCondition=0
  Delay1 : Delay  DelayLength=1  InitialCondition=0
  Delay2 : Delay  DelayLength=1  InitialCondition=0
  Demux1 : Demux  Outputs=3
  MATLAB Function : MATLAB Function  TreatAsAtomicUnit=on
  x : Outport
  y : Outport  Port=2
  z : Outport  Port=3
  wires:
  In1/1 -> Bus Selector/1
  MATLAB Function/2(y) -> y/1
  Constant4/1 -> MATLAB Function/1(depth)
  Delay1/1 -> MATLAB Function/5(act_y)
  Demux1/1 -> Delay/1
  Bus Selector/1 -> Demux1/1  "<Filtered Position>"
  Delay2/1 -> MATLAB Function/6(act_z)
  Delay/1 -> MATLAB Function/4(act_x)
  Constant6/1 -> MATLAB Function/3(pass_height)
  Constant5/1 -> MATLAB Function/2(length)
  Demux1/3 -> Delay2/1
  MATLAB Function/1(x) -> x/1
  Demux1/2 -> Delay1/1
  MATLAB Function/3(z) -> z/1

== system AUV_Model/Translational Reference/Pillar Scanner Logic ==
  note: This logic takes in some dam parameters and the actual position of the robot (provided by the dynamic solver) and updates the reference position to make the robot move along the pillar. 11/2/2024 Thomas
  Act_xyz : Inport
  Bus Selector : BusSelector  OutputSignals=Filtered Position
  Constant1 : Constant  Value=30
  Constant4 : Constant  Value=10
  Constant6 : Constant  Value=5
  Delay : Delay  DelayLength=1  InitialCondition=0
  Delay1 : Delay  DelayLength=1  InitialCondition=0
  Delay2 : Delay  DelayLength=1  InitialCondition=0
  Demux1 : Demux  Outputs=3
  MATLAB Function : MATLAB Function  TreatAsAtomicUnit=on
  x : Outport
  y : Outport  Port=2
  z : Outport  Port=3
  target_angle : Outport  Port=4
  wires:
  Act_xyz/1 -> Bus Selector/1
  MATLAB Function/2(y) -> y/1
  Constant4/1 -> MATLAB Function/2(diameter)
  Delay1/1 -> MATLAB Function/5(act_y)
  Demux1/1 -> Delay/1
  Bus Selector/1 -> Demux1/1  "<Filtered Position>"
  Delay2/1 -> MATLAB Function/6(act_z)
  Delay/1 -> MATLAB Function/4(act_x)
  Constant6/1 -> MATLAB Function/3(pass_height)
  Demux1/3 -> Delay2/1
  MATLAB Function/1(x) -> x/1
  Demux1/2 -> Delay1/1
  MATLAB Function/3(z) -> z/1
  MATLAB Function/4(target_angle) -> target_angle/1
  Constant1/1 -> MATLAB Function/1(depth)

== system AUV_Model/Translational Reference/Signal Builder ==
  Demux : Demux  Tag=STV Demux  Outputs=1
      settings: DisplayOption=none
  FromWs : FromWorkspace  Tag=STV FromWs  VariableName=tuvar
      SigBuilderData=|
      | common.afterFinalStr = 'Extrapolate'
      | common.sampleTime = 0
      | dataSet.timeRange = [0 300]
      | dataSet.name = 'Group 1'
      | sbobj.Groups.Name = 'Group 1'
      | sbobj.Groups.Signals.Name = 'Signal 2'
      | sbobj.Groups.Signals.XData = [0 9 9 16 16 300]
      | sbobj.Groups.Signals.YData = [0.096 0.096 0.2 0.2 0 0]
      | sbobj.Groups.TimeRange = [0 300]
  Signal 2 : Outport  Tag=STV Outport  VectorParamsAs1DForOutWhenUnconnected=off
  wires:
  FromWs/1 -> Demux/1
  Demux/1 -> Signal 2/1

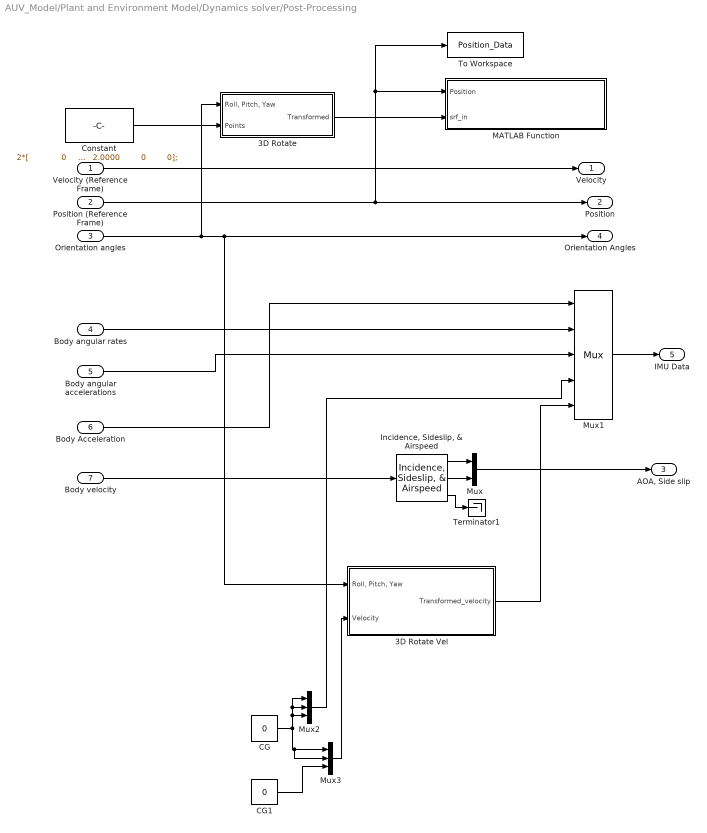
== system AUV_Model/Plant and Environment Model/Dynamics solver/Post-Processing ==
  Velocity (Reference Frame) : Inport
  Position (Reference Frame) : Inport  Port=2
  Orientation angles : Inport  Port=3
  Body angular rates : Inport  Port=4
  Body angular accelerations : Inport  Port=5
  Body Acceleration : Inport  Port=6
  Body velocity : Inport  Port=7
  "3D Rotate " : Subsystem
  3D Rotate Vel : Subsystem
  CG : Constant  Value=0
  CG1 : Constant  Value=0
  Constant : Constant  Value=|
      | 2*[              0         0         0
      |     2.0000         0         0
      |     2.0000    0.4000         0
      |          0    0.4000         0
      |          0         0         0
      |          0         0    0.4000
      |     2.0000         0    0.4000
      |     2.0000    0.4000    0.4000
      |          0    0.4000    0.4000
      |          0         0    0.4000
      |          0    0.4000    0.4000
      |          0    0.4000         0
      |     2.0000    0.4000         0
      |     2.0000    0.4000    0.4000
      |     2.0000         0    0.4000
      |     2.0000         0         0];
  "Incidence, Sideslip, & Airspeed" : aerolibasang/Incidence, Sideslip, & Airspeed
  MATLAB Function : MATLAB Function  TreatAsAtomicUnit=on  SystemSampleTime=0.05
  Mux : Mux  Inputs=2
  Mux1 : Mux  Inputs=5
  Mux2 : Mux  Inputs=3
  Mux3 : Mux  Inputs=3
  Terminator1 : Terminator
  To Workspace : ToWorkspace  VariableName=Position_Data  SampleTime=-1
  Velocity : Outport  VectorParamsAs1DForOutWhenUnconnected=off
  " Position" : Outport  Port=2  VectorParamsAs1DForOutWhenUnconnected=off
  "AOA, Side slip" : Outport  Port=3  VectorParamsAs1DForOutWhenUnconnected=off
  Orientation Angles : Outport  Port=4  VectorParamsAs1DForOutWhenUnconnected=off
  IMU Data : Outport  Port=5  VectorParamsAs1DForOutWhenUnconnected=off
  wires:
  Body angular accelerations/1 -> Mux1/3
  "Incidence, Sideslip, & Airspeed"/2 -> Mux/2
  Body velocity/1 -> "Incidence, Sideslip, & Airspeed"/1
  "Incidence, Sideslip, & Airspeed"/1 -> Mux/1
  Body angular rates/1 -> Mux1/2
  CG/1 -> Mux2/3, Mux2/2, Mux2/1, Mux3/2, Mux3/1
  3D Rotate Vel/1("Transformed_velocity ") -> Mux1/5
  Mux2/1 -> Mux1/4
  Position (Reference Frame)/1 -> To Workspace/1, MATLAB Function/1(Position), " Position"/1
  Mux/1 -> "AOA, Side slip"/1
  CG1/1 -> Mux3/3
  Mux3/1 -> 3D Rotate Vel/2(Velocity)
  Body Acceleration/1 -> Mux1/1
  Velocity (Reference Frame)/1 -> Velocity/1
  Orientation angles/1 -> 3D Rotate Vel/1("Roll, Pitch, Yaw"), Orientation Angles/1, "3D Rotate "/1("Roll, Pitch, Yaw")
  Mux1/1 -> IMU Data/1
  Constant/1 -> "3D Rotate "/2(Points)
  "3D Rotate "/1("Transformed ") -> MATLAB Function/2(srf_in)
  "Incidence, Sideslip, & Airspeed"/3 -> Terminator1/1

== system AUV_Model/Plant and Environment Model/Dynamics solver/Turn Control ==
  note: This block serves to control the robots turning provided a target angle.
  target_angle : Inport
  Constant : Constant
  Delay : Delay  DelayLength=1  InitialCondition=0
  MATLAB Function1 : MATLAB Function  TreatAsAtomicUnit=on
  Mux : Mux  Inputs=3
  Product : Product
  angle : Outport
  wires:
  target_angle/1 -> MATLAB Function1/2(target_angle)
  Constant/1 -> Product/1
  Delay/1 -> MATLAB Function1/1(actual_angle), Product/2
  MATLAB Function1/1(angle) -> Delay/1
  Product/1 -> Mux/3
  Mux/1 -> angle/1

== system AUV_Model/Plant and Environment Model/Environmental Forces & Moments/Hydrodynamic Forces ==
  "Submarine Velocity (Body Axis) " : Inport
  "AOA, Side Slip" : Inport  Port=2
  Hydrodynamic Forces - Accurate : Subsystem  VariantControl=c==1
  Hydrodynamic Forces - Basic : Subsystem  VariantControl=c==0
  "Force due to Lift, Drag" : Outport  VectorParamsAs1DForOutWhenUnconnected=off

== system AUV_Model/Plant and Environment Model/Environmental Forces & Moments/Hydrostatic Forces ==
  In1 : Inport
  Constant : Constant
  Environment Model : Subsystem  mask{ro=997, V=0.01, M=10, a=0, b=0, c=0}
      mask prompts: ro "Density of Water"; V "Volume of Submarine"; M "Mass of Submarine"; a "X Distance between CG and CB"; b "Y Distance between CG and CB"; c "Z Distance between CG and CB"
      mask DialogControl DescTextVar Prompt: Enter the Submarine related Parameters
      mask DialogControl Container3 Prompt: Distance between CG and Center of Buoyancy
  Hydrostatic Force : Outport  VectorParamsAs1DForOutWhenUnconnected=off
  Hydrostatic Moment : Outport  Port=2  VectorParamsAs1DForOutWhenUnconnected=off
  wires:
  Constant/1 -> Environment Model/1("Fraction submerged ")
  Environment Model/2(Moment due to Weight and Buoyancy) -> Hydrostatic Moment/1
  Environment Model/1(Forces due to Weight and Buoyancy) -> Hydrostatic Force/1
  In1/1 -> Environment Model/2(Orientation Angles)

== system AUV_Model/Plant and Environment Model/Propulsion Forces & Moments/Force and moments due to Thrust ==
  Thrust Inputs : Inport
  "Thrust to Propulsion " : Subsystem
  Propulsion Force : Outport  VectorParamsAs1DForOutWhenUnconnected=off
  Propulsion Moment : Outport  Port=2  VectorParamsAs1DForOutWhenUnconnected=off
  wires:
  "Thrust to Propulsion "/2(Propulsion Moment) -> Propulsion Moment/1
  Thrust Inputs/1 -> "Thrust to Propulsion "/1(Thrust Inputs)
  "Thrust to Propulsion "/1(Propulsion Force) -> Propulsion Force/1

== system AUV_Model/Plant and Environment Model/Propulsion Forces & Moments/Input commands to Thrust ==
  Thrust Control Inputs : Inport
  Demux : Demux  Outputs=3
  Input Commands to PWM : Subsystem
  "PWM Signals to Thrust " : Subsystem
  Thrust values : Outport  VectorParamsAs1DForOutWhenUnconnected=off
  wires:
  Input Commands to PWM/1(Px1) -> "PWM Signals to Thrust "/1(PWM Signal Px1)
  Input Commands to PWM/3(Py1) -> "PWM Signals to Thrust "/3(PWM Signal Py1)
  Demux/1 -> Input Commands to PWM/1(X Thruster)  "X Thrust Input"
  Demux/3 -> Input Commands to PWM/3(Z Thruster)  "Z Thrust Input"
  Input Commands to PWM/4(Py2) -> "PWM Signals to Thrust "/4(PWM Signal Py2)
  Demux/2 -> Input Commands to PWM/2(Y Thruster)  "Y Thrust Input"
  Input Commands to PWM/2(Px2) -> "PWM Signals to Thrust "/2(PWM Signal Px2)
  Input Commands to PWM/5(Pz) -> "PWM Signals to Thrust "/5(PWM Signal Pz)
  "PWM Signals to Thrust "/1(Thrust (N)) -> Thrust values/1
  Thrust Control Inputs/1 -> Demux/1

== system AUV_Model/Sensor data and State Estimation/System With Noise/ Sensor (IMU) ==
  IMU Inputs : Inport
  Bus Creator : BusCreator  Inputs=2
  Bus Selector : BusSelector  OutputSignals=IMU Data
  Demux : Demux  Outputs=5
  Three-axis Inertial Measurement Unit : aerolibnav/Three-axis Inertial Measurement Unit  units=Metric (MKS)  imu=[0 0 0]  i_Ts=0  dtype_a=on  w_a=190  z_a=0.707  a_sf_cc=[1 0 0; 0 1 0; 0 0 1]  a_bias=[0 0 0]  a_sat="[-inf  -inf  -inf  inf inf inf]"  dtype_g=on  w_g=190  z_g=0.707  g_sf_cc=[1 0 0; 0 1 0; 0 0 1]  g_bias=[0 0 0]  g_sens=[0 0 0]  g_sat="[-inf  -inf  -inf  inf inf inf]"  i_rand=on  i_seeds=[23093 23094 23095 23096 23097 23098]  i_pow=[0.00001 0.00001 0.00001 0.00001 0.00001 0.00001]
  IMU Measurements : Outport  VectorParamsAs1DForOutWhenUnconnected=off
  wires:
  Three-axis Inertial Measurement Unit/1 -> Bus Creator/1  "IMU Measured Acceleration"
  Demux/2 -> Three-axis Inertial Measurement Unit/2
  Demux/4 -> Three-axis Inertial Measurement Unit/4
  Demux/5 -> Three-axis Inertial Measurement Unit/5
  Demux/3 -> Three-axis Inertial Measurement Unit/3
  Demux/1 -> Three-axis Inertial Measurement Unit/1
  Three-axis Inertial Measurement Unit/2 -> Bus Creator/2  "IMU Measured Body Rates"
  IMU Inputs/1 -> Bus Selector/1
  Bus Selector/1 -> Demux/1  "<IMU Data>"
  Bus Creator/1 -> IMU Measurements/1

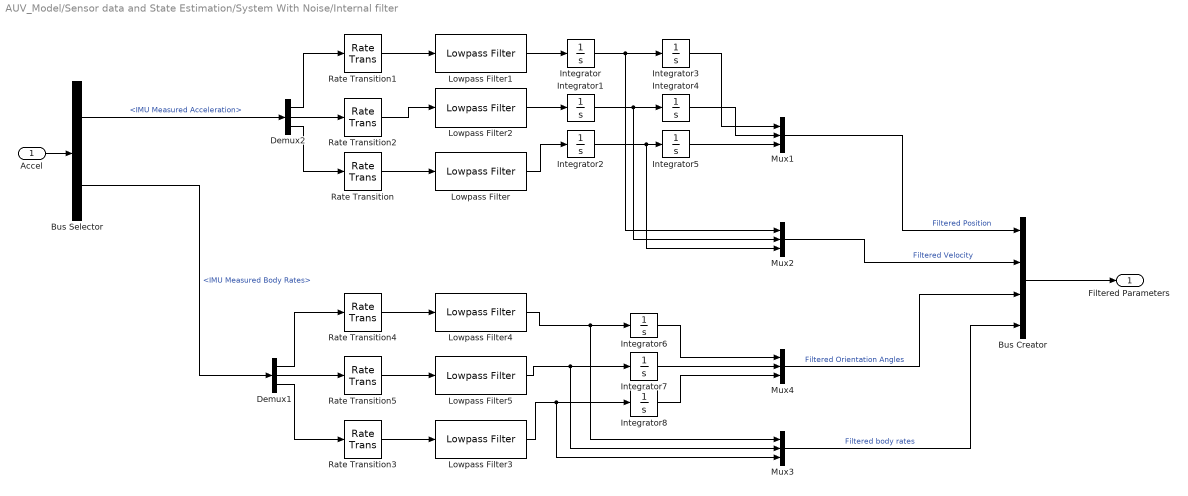
== system AUV_Model/Sensor data and State Estimation/System With Noise/Internal filter ==
  Accel : Inport
  Bus Creator : BusCreator  Inputs=4
  Bus Selector : BusSelector  OutputSignals=IMU Measured Acceleration,IMU Measured Body Rates
  Demux1 : Demux  Outputs=3
  Demux2 : Demux  Outputs=3
  Integrator{,1..8} (9 alike) : Integrator
  Lowpass Filter{,1..5} (6 alike) : dspfdesign/Lowpass Filter  FilterType=FIR  DesignForMinimumOrder=on  FilterOrder=50  PassbandFrequency=1/100  StopbandFrequency=45  PassbandRipple=0.1  StopbandAttenuation=80  SampleRateMode=Specify on dialog  SampleRate=100  SimulateUsing=Interpreted execution  roundingMode=Floor  coeffsDataTypeStr=fixdt(1,16)
  Mux{1..4} (4 alike) : Mux  Inputs=3
  Rate Transition{,1..5} (6 alike) : RateTransition  OutPortSampleTime=0.01
  Filtered Parameters : Outport  VectorParamsAs1DForOutWhenUnconnected=off
  wires:
  Rate Transition5/1 -> Lowpass Filter5/1
  Rate Transition4/1 -> Lowpass Filter4/1
  Demux1/1 -> Rate Transition4/1
  Lowpass Filter3/1 -> Mux3/3, Integrator8/1
  Demux1/2 -> Rate Transition5/1
  Lowpass Filter5/1 -> Mux3/2, Integrator7/1
  Lowpass Filter4/1 -> Mux3/1, Integrator6/1
  Integrator6/1 -> Mux4/1
  Rate Transition3/1 -> Lowpass Filter3/1
  Integrator8/1 -> Mux4/3
  Demux1/3 -> Rate Transition3/1
  Integrator7/1 -> Mux4/2
  Accel/1 -> Bus Selector/1
  Bus Selector/1 -> Demux2/1  "<IMU Measured Acceleration>"
  Bus Selector/2 -> Demux1/1  "<IMU Measured Body Rates>"
  Mux4/1 -> Bus Creator/3  "Filtered Orientation Angles"
  Mux3/1 -> Bus Creator/4  "Filtered body rates"
  Bus Creator/1 -> Filtered Parameters/1
  Integrator2/1 -> Integrator5/1, Mux2/3
  Integrator/1 -> Mux2/1, Integrator3/1
  Mux2/1 -> Bus Creator/2  "Filtered Velocity"
  Mux1/1 -> Bus Creator/1  "Filtered Position"
  Lowpass Filter/1 -> Integrator2/1
  Demux2/2 -> Rate Transition2/1
  Rate Transition1/1 -> Lowpass Filter1/1
  Integrator4/1 -> Mux1/2
  Demux2/3 -> Rate Transition/1
  Lowpass Filter2/1 -> Integrator1/1
  Lowpass Filter1/1 -> Integrator/1
  Demux2/1 -> Rate Transition1/1
  Integrator5/1 -> Mux1/3
  Integrator1/1 -> Integrator4/1, Mux2/2
  Rate Transition/1 -> Lowpass Filter/1
  Integrator3/1 -> Mux1/1
  Rate Transition2/1 -> Lowpass Filter2/1

== system AUV_Model/Plant and Environment Model/Dynamics solver/Post-Processing/3D Rotate  ==
  "Roll, Pitch, Yaw" : Inport
  Points : Inport  Port=2
  Gain : Gain
  Matrix Multiply : Product  Multiplication=Matrix(*)
  Rotation Angles to Direction Cosine Matrix : sharedtransform/Rotation Angles to Direction Cosine Matrix  rotationOrder=XYZ  aMode=aMode
  Transpose : Math  Operator=transpose  SignedPower=on
  "Transformed " : Outport  VectorParamsAs1DForOutWhenUnconnected=off
  wires:
  Matrix Multiply/1 -> "Transformed "/1
  Rotation Angles to Direction Cosine Matrix/1 -> Transpose/1
  Points/1 -> Matrix Multiply/1
  "Roll, Pitch, Yaw"/1 -> Gain/1
  Transpose/1 -> Matrix Multiply/2
  Gain/1 -> Rotation Angles to Direction Cosine Matrix/1

== system AUV_Model/Plant and Environment Model/Dynamics solver/Post-Processing/3D Rotate Vel ==
  "Roll, Pitch, Yaw" : Inport
  Velocity : Inport  Port=2
  Gain : Gain
  Matrix Multiply : Product  Multiplication=Matrix(*)
  Rotation Angles to Direction Cosine Matrix : sharedtransform/Rotation Angles to Direction Cosine Matrix  rotationOrder=XYZ  aMode=aMode
  Transpose : Math  Operator=transpose  SignedPower=on
  "Transformed_velocity " : Outport  VectorParamsAs1DForOutWhenUnconnected=off
  wires:
  Matrix Multiply/1 -> "Transformed_velocity "/1
  Rotation Angles to Direction Cosine Matrix/1 -> Transpose/1
  Velocity/1 -> Matrix Multiply/2
  "Roll, Pitch, Yaw"/1 -> Gain/1
  Transpose/1 -> Matrix Multiply/1
  Gain/1 -> Rotation Angles to Direction Cosine Matrix/1

== system AUV_Model/Plant and Environment Model/Environmental Forces & Moments/Hydrodynamic Forces/Hydrodynamic Forces - Accurate ==
  note: Source of Equations:
      | Submarine Dynamic Modeling, by
      | Dr Peter Ridley Julien Fontan and Dr Peter Corke
      |
      | Part: Hydrodynamic forces and moments
  "Submarine Velocity (Body Axis) " : Inport
  "AOA, Side Slip" : Inport  Port=2
  Force Exerted due to Drag (Body Axis) : Subsystem
  Force Exerted due to Lift (Body Axis) : Subsystem
  Sum : Sum
  "Force due to Lift, Drag" : Outport  VectorParamsAs1DForOutWhenUnconnected=off
  wires:
  Force Exerted due to Drag (Body Axis)/1(Drag Forces in Body Axis) -> Sum/1
  Force Exerted due to Lift (Body Axis)/1(Lift Forces in Body Axis) -> Sum/2
  "AOA, Side Slip"/1 -> Force Exerted due to Drag (Body Axis)/2(AOA and Side Slip), Force Exerted due to Lift (Body Axis)/2(AOA and Side Slip)
  "Submarine Velocity (Body Axis) "/1 -> Force Exerted due to Lift (Body Axis)/1(Marine Velocities in Body Axis), Force Exerted due to Drag (Body Axis)/1(Marine Velocities in Body Axis)
  Sum/1 -> "Force due to Lift, Drag"/1

== system AUV_Model/Plant and Environment Model/Environmental Forces & Moments/Hydrodynamic Forces/Hydrodynamic Forces - Basic ==
  "Submarine Velocity (Body Axis) " : Inport
  "AOA, Side Slip" : Inport  Port=2
  Force Exerted due to Drag (Body Axis) : Subsystem
  Force Exerted due to Lift (Body Axis) : Subsystem
  Sum : Sum
  "Force due to Lift, Drag" : Outport  VectorParamsAs1DForOutWhenUnconnected=off
  wires:
  Force Exerted due to Drag (Body Axis)/1(Drag Forces in Body Axis) -> Sum/1
  Force Exerted due to Lift (Body Axis)/1(Lift Forces in Body Axis) -> Sum/2
  "AOA, Side Slip"/1 -> Force Exerted due to Drag (Body Axis)/2(AOA and Side Slip), Force Exerted due to Lift (Body Axis)/2(AOA and Side Slip)
  "Submarine Velocity (Body Axis) "/1 -> Force Exerted due to Lift (Body Axis)/1(Marine Velocities in Body Axis), Force Exerted due to Drag (Body Axis)/1(Marine Velocities in Body Axis)
  Sum/1 -> "Force due to Lift, Drag"/1

== system AUV_Model/Plant and Environment Model/Environmental Forces & Moments/Hydrostatic Forces/Environment Model ==
  "Fraction submerged " : Inport
  Orientation Angles : Inport  Port=2
  3D Rotate Drag : Subsystem
  Constant : Constant  Value=-ro*9.81*V
  Constant1 : Constant  Value=0
  Constant2 : Constant  Value=+M*9.81
  Constant3 : Constant  Value=[a;b;c]
  Cross Product : vrlib/Utilities/Cross Product
  Multiply : Product
  Mux : Mux  Inputs=3
  Mux1 : Mux  Inputs=3
  Sum : Sum
  Forces due to Weight and Buoyancy : Outport  VectorParamsAs1DForOutWhenUnconnected=off
  Moment due to Weight and Buoyancy : Outport  Port=2  VectorParamsAs1DForOutWhenUnconnected=off
  wires:
  Cross Product/1 -> Moment due to Weight and Buoyancy/1
  Constant3/1 -> Cross Product/1
  "Fraction submerged "/1 -> Multiply/2
  Mux/1 -> Sum/2
  Multiply/1 -> Mux/3
  Mux1/1 -> Sum/1, Cross Product/2
  Constant/1 -> Multiply/1
  Constant1/1 -> Mux/1, Mux/2, Mux1/2, Mux1/1
  Constant2/1 -> Mux1/3
  Sum/1 -> 3D Rotate Drag/1(Force)
  Orientation Angles/1 -> 3D Rotate Drag/2("Roll, Pitch, Yaw")
  3D Rotate Drag/1("Transformed_Force ") -> Forces due to Weight and Buoyancy/1
